simulink model "Tanques_quick_start"  (R2014a)
settings: Solver=ode1  StartTime=0.0  StopTime=200  FixedStep=0.1  RelTol=1e-3
PostLoadFcn:
  | qc_set_target_type(getConfigSet(bdroot, 'QUARC Default Target Configuration'));
values from neighbouring files (symbols this model uses):
  a = sys.a    [Init_SS.m]    (also in test.m)
  b = sys.b    [Init_SS.m]    (also in test.m)
  c = sys.c    [Init_SS.m]    (also in test.m)
  k = [K(2) K(3)]    [Init_SS.m]    (also in test.m = [0.9 0.9])
  ke = K(1)    [Init_SS.m]
  L = acker(a', c', polos_observer)'    [Init_SS.m]    (also in Observer.m = [1.1; 0.2]; test.m = acker(a', c', k)')
undefined symbols (not defined in the file or in its folder): HIL
libraries: quarc_library x3, simulink x1, commrandsrc2 x1
PauseFcn:
  | get_amplitude_and_period(amin, amax, pmin, pmax)
settings Model: SimulationMode=external  ExtModeTrigDuration=30000  Creator=MLevis  LastModifiedBy=Aluno IC
settings SolverCC: PositivePriorityOrder=on
settings DataIOCC: SignalLoggingSaveFormat=ModelDataLogs
settings OptimizationCC: ExpressionDepthLimit=2147483647  InitFltsAndDblsToZero=on
settings DebuggingCC: SaveWithParameterizedLinksMsg=none  UnderspecifiedInitializationDetection=Classic  MultiTaskDSMMsg=warning  MultiTaskCondExecSysMsg=none  FcnCallInpInsideContextMsg=UseLocalSettings  StateNameClashWarn=warning
settings RTWCC: SystemTargetFile=quarc_win64.tlc  TemplateMakefile=quarc_default_tmf  Description=QUARC Win64 Target  ProcessScript=quarc_win64_make_rtw_hook
settings STFCustomTargetCC: CPPClassGenCompliant=on
settings GRTTargetCC: ParMdlRefBuildCompliant=off  CompOptLevelCompliant=off  CombineOutputUpdateFcns=off  MatFileLogging=off  GRTInterface=on  ExtMode=on  ExtModeMexFile=quarc_comm

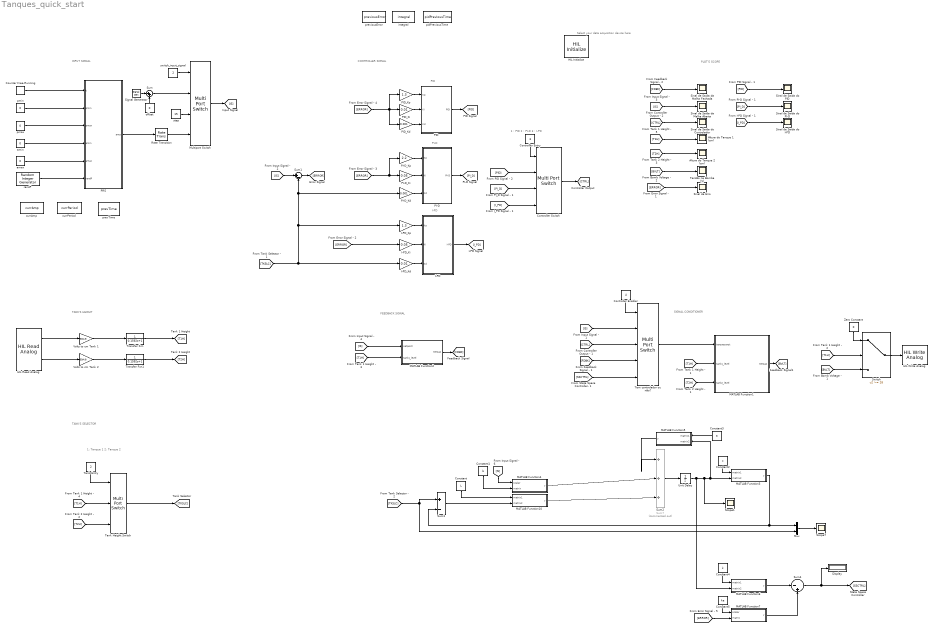
== system Tanques_quick_start ==
  note: INPUT SIGNAL
  note: Select your data acquisition device here
  note: TANK'S HEIGHT
  note: FEEDBACK SIGNAL
  note: CONTROLLER SIGNAL
  note: SIGNAL CONDITIONER
  note: PLOT'S SCOPE
  note: 1 : PID
      | 2 : PI-D
      | 3 : I-PD
  note: I-PD
  note: PI-D
  note: PID
  note: 1: Tanque 1
      | 2: Tanque 2
  note: TANK'S SELECTOR
  Altura do Tanque 1 (cm) : Scope
      settings: TimeRange=200  YMin=-5.5  YMax=30  SaveName=Tank_1_Height_Data
  Altura do Tanque 2 (cm) : Scope
      settings: TimeRange=120  YMin=0  YMax=30  SaveName=Tank_2_Height_Data
  Constant : Constant  Value=L  VectorParams1D=off
  Constant1 : Constant  Value=b  VectorParams1D=off
  Constant2 : Constant  Value=c  VectorParams1D=off
  Constant3 : Constant  Value=a  VectorParams1D=off
  Constant4 : Constant  Value=k  VectorParams1D=off
  Constant5 : Constant  Value=ke  VectorParams1D=off
  "Controller Enabler " : Constant  Value=4
  Controller Entry : Constant  Value=3
  Controller Switch : MultiPortSwitch
  Counter Free-Running : simulink/Sources/Counter Free-Running  NumBits=16  tsamp=1
  Display : Display
  HIL Initialize : quarc_library/Data Acquisition/Generic/Configuration/HIL Initialize  object_name=HIL-1  board_type=q2_usb  board_number=0  board_options=d0=digital;d1=digital;led=auto;update_rate=normal;decimation=1  exclusive=off  active=off  hardware_clocks=[0]  clock_modes=[]  initial_clock_frequencies=[]  set_clock_params_at_start=off  set_clock_params_at_switch_in=off  set_clock_frequencies_at_start=off  set_clock_frequencies_at_switch_in=off  analog_input_channels=[0:1]  analog_input_maximums=10  analog_input_minimums=-10  set_analog_input_params_at_start=on  set_analog_input_params_at_switch_in=off  analog_output_channels=[0:1]  analog_output_maximums=10  analog_output_minimums=-10  initial_analog_outputs=[0]  final_analog_outputs=[0]  watchdog_analog_outputs=0  set_analog_output_params_at_start=on  set_analog_output_params_at_switch_in=off  set_analog_outputs_at_start=on  set_analog_outputs_at_switch_in=off  set_analog_outputs_at_terminate=on  set_analog_outputs_at_switch_out=off  set_analog_outputs_on_watchdog=off  digital_input_channels=[]  digital_output_channels=[]  digital_output_configuration=[]  initial_digital_outputs=[1]  final_digital_outputs=[1]  watchdog_digital_outputs=[1]  set_digital_output_params_at_start=off  set_digital_output_params_at_switch_in=off  set_digital_outputs_at_start=on  set_digital_outputs_at_switch_in=off  set_digital_outputs_at_terminate=on  set_digital_outputs_at_switch_out=off  set_digital_outputs_on_watchdog=off  encoder_channels=[0:1]  quadrature=[4]  encoder_filter_frequency=[]  initial_encoder_counts=[0]  set_encoder_params_at_start=on  set_encoder_params_at_switch_in=off  set_encoder_counts_at_start=on  set_encoder_counts_at_switch_in=off  pwm_channels=[]  pwm_modes=[0]  pwm_frequency=1/0.020  pwm_configuration=[]  pwm_alignment=[]  pwm_polarity=[]  pwm_leading_deadband=[]  pwm_trailing_deadband=[]  initial_pwm_outputs=[0]  final_pwm_outputs=[0]  watchdog_pwm_outputs=[0]  set_pwm_params_at_start=on  set_pwm_params_at_switch_in=off  set_pwm_outputs_at_start=on  set_pwm_outputs_at_switch_in=off  set_pwm_outputs_at_terminate=on  set_pwm_outputs_at_switch_out=off  set_pwm_outputs_on_watchdog=off  other_output_channels=[]  initial_other_outputs=[]  final_other_outputs=[]  watchdog_other_outputs=[]  set_other_outputs_at_start=off  set_other_outputs_at_switch_in=off  set_other_outputs_at_terminate=off  set_other_outputs_at_switch_out=off  set_other_outputs_on_watchdog=off
  HIL Read Analog : quarc_library/Data Acquisition/Generic/Immediate I//O/HIL Read Analog  object_name=HIL-1  channels=[0:1]  sample_time=qc_get_step_size  active=on  vector_output=off
  HIL Write Analog : quarc_library/Data Acquisition/Generic/Immediate I//O/HIL Write Analog  object_name=HIL-1  channels=0  sample_time=-1  active=off  vector_input=off
  I-PD : Subsystem
  I-PD_Kd : Gain  Gain=0.01
  I-PD_Ki : Gain  Gain=0.05
  I-PD_Kp : Gain  Gain=1.3
  MATLAB Function1 : MATLAB Function  TreatAsAtomicUnit=on
  MATLAB Function10 : MATLAB Function  TreatAsAtomicUnit=on
  MATLAB Function2 : MATLAB Function  TreatAsAtomicUnit=on
  MATLAB Function3 : MATLAB Function  TreatAsAtomicUnit=on
  MATLAB Function4 : MATLAB Function  TreatAsAtomicUnit=on
  MATLAB Function5 : MATLAB Function  TreatAsAtomicUnit=on
  MATLAB Function6 : MATLAB Function  TreatAsAtomicUnit=on
  MATLAB Function7 : MATLAB Function  TreatAsAtomicUnit=on
  Multiport Switch : MultiPortSwitch
  Mux : Mux  Inputs=2
  PI-D : Subsystem
  PI-D_Kd : Gain  Gain=0.001
  "PI-D_Ki " : Gain  Gain=0.05
  PI-D_Kp : Gain  Gain=2.2
  PID : Subsystem
  PID_Kd : Gain  Gain=0.001
  PID_Ki : Gain  Gain=0.01
  PID_Kp : Gain  Gain=1.3
  PRS : MATLAB Function  TreatAsAtomicUnit=on
  Rate Transition : RateTransition  OutPortSampleTime=0.1
  Scope1 : Scope
      settings: YMin=0  YMax=50
  Scope7 : Scope
      settings: YMin=0  YMax=50  SaveName=ScopeData6
  Signal Generator : SignalGenerator  Amplitude=15  Frequency=6.2832  Units=rad/sec
  Sinal de Erro : Scope
      settings: TimeRange=200  YMin=-3  YMax=15  SaveName=tensao1
  Sinal de Saída da Malha Aberta : Scope
      settings: TimeRange=200  YMin=9  YMax=15  SaveName=ScopeData3
  Sinal de Saída da Malha Fechada : Scope
      settings: YMin=9.25  YMax=14.75  SaveName=ScopeData7
  Sinal de Saída do Controlador : Scope
      settings: TimeRange=200  YMin=9  YMax=15  SaveName=ScopeData4
  Sinal de Saída do I-PD : Scope
      settings: YMin=-7.5  YMax=32.5  SaveName=I_PD_Data
  Sinal de Saída do PI-D : Scope
      settings: TimeRange=120  YMax=40  SaveName=PI_D_Data
  Sinal de Saída do PID : Scope
      settings: TimeRange=200  YMin=-2.5  YMax=32.5  SaveName=PID_Data
  Sum : Sum  Inputs=|++
  Sum1 : Sum  Inputs=|+-
  Sum2 : Sum  Inputs=|+++
  Sum3 : Sum  Inputs=|+-
  Sum4 : Sum  Inputs=|-+
  Sum7 : Sum  Commented=on  Inputs=|+++
  Switch : Switch  Threshold=28
  Tank Entry : Constant  Value=2
  Tank Height Switch : MultiPortSwitch  Inputs=2
  "Tem controlador ou não? " : MultiPortSwitch  Inputs=4
  Tensão na Bomba (V) : Scope
      settings: TimeRange=30  SaveName=tensao
  Transfer Fcn : TransferFcn  Denominator=[0.1592 1]
  Transfer Fcn1 : TransferFcn  Denominator=[0.1592 1]
  Unit Delay : UnitDelay  SampleTime=-1
  "Volts to cm Tank 1 " : Gain  Gain=30/4.8
  Volts to cm Tank 2 : Gain  Gain=30/4.8
  Zero Constant : Constant  Value=0
  amax : Constant  Value=0  OutDataTypeStr=double
  amin : Constant  Value=0  OutDataTypeStr=double
  currAmp : DataStoreMemory  DataStoreName=currAmp  ReadBeforeWriteMsg=warning  WriteAfterWriteMsg=warning  WriteAfterReadMsg=warning  OutDataTypeStr=double
  currPeriod : DataStoreMemory  DataStoreName=currPeriod  ReadBeforeWriteMsg=warning  WriteAfterWriteMsg=warning  WriteAfterReadMsg=warning  OutDataTypeStr=uint16
  integral : DataStoreMemory  DataStoreName=integral  ReadBeforeWriteMsg=warning  WriteAfterWriteMsg=warning  WriteAfterReadMsg=warning  OutDataTypeStr=double
  offset : Constant  Value=0
  pidPreviousTime : DataStoreMemory  DataStoreName=pidPreviousTime  ReadBeforeWriteMsg=warning  WriteAfterWriteMsg=warning  WriteAfterReadMsg=warning  OutDataTypeStr=double
  pmax : Constant  Value=0  OutDataTypeStr=uint16
  pmin : Constant  Value=0  OutDataTypeStr=uint16
  prevTime : DataStoreMemory  DataStoreName=prevTime  ReadBeforeWriteMsg=warning  WriteAfterWriteMsg=warning  WriteAfterReadMsg=warning  OutDataTypeStr=uint16
  previousError : DataStoreMemory  DataStoreName=previousError  ReadBeforeWriteMsg=warning  WriteAfterWriteMsg=warning  WriteAfterReadMsg=warning  OutDataTypeStr=double
  randP : commrandsrc2/Random Integer Generator  mul=5  seed=37  Ts=1  frameBased=off  sampPerFrame=1  orient=off  outDataType=uint16
  step : Constant  Value=15
  switch_input_signal : Constant  Value=2
  wires:
  HIL Read Analog/1 -> "Volts to cm Tank 1 "/1
  "Volts to cm Tank 1 "/1 -> Transfer Fcn/1
  Transfer Fcn1/1 -> [T2H]
  Volts to cm Tank 2/1 -> Transfer Fcn1/1
  HIL Read Analog/2 -> Volts to cm Tank 2/1
  switch_input_signal/1 -> Multiport Switch/1
  step/1 -> Multiport Switch/3
  Signal Generator/1 -> Sum/1
  offset/1 -> Sum/2
  Sum/1 -> Multiport Switch/2
  Counter Free-Running/1 -> PRS/1(t)
  pmin/1 -> PRS/2(pmin)
  pmax/1 -> PRS/3(pmax)
  amin/1 -> PRS/4(amin)
  amax/1 -> PRS/5(amax)
  randP/1 -> PRS/6(randP)
  PRS/1(amp) -> Rate Transition/1
  Zero Constant/1 -> Switch/1
  Switch/1 -> HIL Write Analog/1
  Rate Transition/1 -> Multiport Switch/4
  Multiport Switch/1 -> [IS]
  Transfer Fcn/1 -> [T1H]
  "Controller Enabler "/1 -> "Tem controlador ou não? "/1
  "Tem controlador ou não? "/1 -> MATLAB Function1/1(tensaoconst)
  [T1H] -> MATLAB Function2/2(tank1_level)
  [T1H] -> MATLAB Function1/2(tank1_level)
  [T1H] -> Switch/2
  [T2H] -> MATLAB Function1/3(tank2_level)
  [IS] -> "Tem controlador ou não? "/2
  [IS] -> Sinal de Saída da Malha Aberta/1
  [IS] -> MATLAB Function2/1(setpoint)
  Controller Switch/1 -> [CTRL]
  [CTRL] -> "Tem controlador ou não? "/3
  MATLAB Function2/1(tensao) -> [FDBK]
  [FDBK] -> "Tem controlador ou não? "/4
  [FDBK] -> Sinal de Saída da Malha Fechada/1
  [T1H] -> Altura do Tanque 1 (cm)/1
  [T2H] -> Altura do Tanque 2 (cm)/1
  MATLAB Function1/1(tensao) -> [BVLT]
  [BVLT] -> Switch/3
  [BVLT] -> Tensão na Bomba (V)/1
  [CTRL] -> Sinal de Saída do Controlador/1
  [ERROR] -> Sinal de Erro/1
  [PID] -> Sinal de Saída do PID/1
  [PI_D] -> Sinal de Saída do PI-D/1
  [I_PD] -> Sinal de Saída do I-PD/1
  PID_Kp/1 -> PID/1(" Kp")
  PID_Kd/1 -> PID/3(Kd)
  PID_Ki/1 -> PID/2(Ki)
  PI-D/1(PI-D) -> [PI_D]
  Sum1/1 -> [ERROR]
  Controller Entry/1 -> Controller Switch/1
  I-PD/1(I-PD) -> [I_PD]
  PID/1(PID) -> [PID]
  [ERROR] -> I-PD_Ki/1
  [ERROR] -> PI-D_Kp/1, "PI-D_Ki "/1
  [ERROR] -> PID_Kd/1, PID_Ki/1, PID_Kp/1
  [PID] -> Controller Switch/2
  [I_PD] -> Controller Switch/4
  [PI_D] -> Controller Switch/3
  PI-D_Kp/1 -> PI-D/1(" Kp")
  PI-D_Kd/1 -> PI-D/3(Kd)
  "PI-D_Ki "/1 -> PI-D/2(" Ki")
  I-PD_Kp/1 -> I-PD/1(" Kp")
  I-PD_Kd/1 -> I-PD/3(Kd)
  I-PD_Ki/1 -> I-PD/2(" Ki")
  [IS] -> Sum1/1
  Constant/1 -> MATLAB Function10/1(matrix1)
  MATLAB Function4/1(y) -> Sum2/2
  [IS] -> MATLAB Function4/1(scalar)
  Constant1/1 -> MATLAB Function4/2(matrix)
  MATLAB Function10/1(y) -> Sum2/3
  MATLAB Function3/1(y) -> Mux/1, Sum3/2
  Constant2/1 -> MATLAB Function3/1(matrix1)
  Constant3/1 -> MATLAB Function5/1(matrix1)
  [TKSLC] -> Mux/2, Sum3/1
  Sum3/1 -> MATLAB Function10/2(matrix2)
  MATLAB Function5/1(y) -> Sum2/1
  Sum2/1 -> Unit Delay/1
  Unit Delay/1 -> MATLAB Function6/2(matrix2), Scope1/1, MATLAB Function3/2(matrix2), MATLAB Function5/2(matrix2)
  Mux/1 -> Scope7/1
  [TKSLC] -> PI-D_Kd/1, Sum1/2, I-PD_Kp/1, I-PD_Kd/1
  Tank Entry/1 -> Tank Height Switch/1
  [T1H] -> Tank Height Switch/2
  [T2H] -> Tank Height Switch/3
  Tank Height Switch/1 -> [TKSLC]
  Constant4/1 -> MATLAB Function6/1(matrix1)
  MATLAB Function6/1(y) -> Sum4/1
  Constant5/1 -> MATLAB Function7/1(scalar)
  MATLAB Function7/1(y) -> Sum4/2
  [ERROR] -> MATLAB Function7/2(matrix)
  Sum4/1 -> Display/1, [SSCTRL]
  [SSCTRL] -> "Tem controlador ou não? "/5

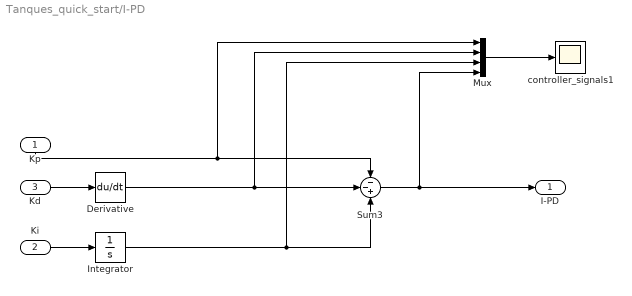
== system Tanques_quick_start/I-PD ==
  " Kp" : Inport
  " Ki" : Inport  Port=2
  Kd : Inport  Port=3
  Derivative : Derivative
  Integrator : Integrator  LimitOutput=on  UpperSaturationLimit=35  LowerSaturationLimit=-1
  Mux : Mux
  Sum3 : Sum  Inputs=--+
  controller_signals1 : Scope
      settings: ShowLegends=on  TimeRange=200  YMin=-10  YMax=150
  I-PD : Outport
  wires:
  Derivative/1 -> Mux/2, Sum3/2
  " Kp"/1 -> Mux/1, Sum3/1
  Sum3/1 -> Mux/4, I-PD/1
  Integrator/1 -> Mux/3, Sum3/3
  Kd/1 -> Derivative/1
  " Ki"/1 -> Integrator/1
  Mux/1 -> controller_signals1/1

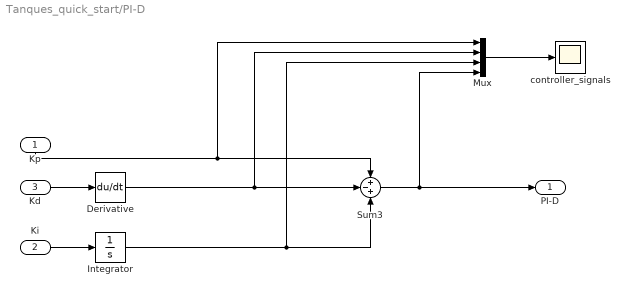
== system Tanques_quick_start/PI-D ==
  " Kp" : Inport
  " Ki" : Inport  Port=2
  Kd : Inport  Port=3
  Derivative : Derivative
  Integrator : Integrator
  Mux : Mux
  Sum3 : Sum  Inputs=+-+
  controller_signals : Scope
      settings: ShowLegends=on  TimeRange=150  YMin=-15  YMax=50
  PI-D : Outport
  wires:
  Derivative/1 -> Mux/2, Sum3/2
  " Kp"/1 -> Mux/1, Sum3/1
  Sum3/1 -> Mux/4, PI-D/1
  Integrator/1 -> Mux/3, Sum3/3
  Kd/1 -> Derivative/1
  " Ki"/1 -> Integrator/1
  Mux/1 -> controller_signals/1

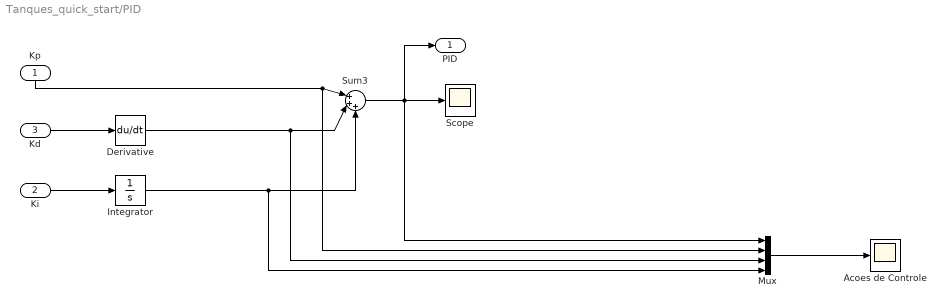
== system Tanques_quick_start/PID ==
  " Kp" : Inport
  Ki : Inport  Port=2
  Kd : Inport  Port=3
  Acoes de Controle : Scope
      settings: ShowLegends=on  TimeRange=200  YMin=-2.5  YMax=32.5  SaveName=ScopeData5
  Derivative : Derivative
  Integrator : Integrator  LimitOutput=on
  Mux : Mux
  Scope : Scope
      settings: ShowLegends=on  TimeRange=90  YMin=10  YMax=47.5  SaveName=ScopeData2
  Sum3 : Sum  Inputs=|+++
  PID : Outport
  wires:
  Derivative/1 -> Mux/3, Sum3/2
  Integrator/1 -> Mux/4, Sum3/3
  " Kp"/1 -> Mux/2, Sum3/1
  Ki/1 -> Integrator/1
  Kd/1 -> Derivative/1
  Sum3/1 -> Mux/1, PID/1, Scope/1
  Mux/1 -> Acoes de Controle/1

== matlab function Tanques_quick_start/MATLAB Function1 ==
  data: tensaoconst input; tensao output; tank1_level input; tank2_level input
function tensao  = trava(tensaoconst, tank1_level, tank2_level)
%#codegen
%Trava para a tensão

if(tensaoconst > 4)
   tensaoconst = 4;
elseif(tensaoconst < -4)
    tensaoconst = -4;
end

%%Trava pro tanque
hmax = 30;

if(tank1_level < 2 && tensaoconst < 0)
    tensaoconst=0;
elseif(-tank1_level+hmax > 5 && -tank1_level+hmax < 6)
    tensaoconst=tensaoconst;
elseif(-tank1_level+hmax > 4 && -tank1_level+hmax < 5)
    tensaoconst=tensaoconst*0.9;
elseif(-tank1_level+hmax > 3 && -tank1_level+hmax < 4)
    tensaoconst=tensaoconst*0.8;
elseif(-tank1_level+hmax > 2 && -tank1_level+hmax< 3)
    tensaoconst=tensaoconst*0.79;
elseif(-tank1_level+hmax > 1 && -tank1_level+hmax < 1.5)
    tensaoconst=tensaoconst*0.70;
elseif(-tank1_level+hmax > 0.5 && -tank1_level+hmax < 0.8)
    tensaoconst=tensaoconst*0.55;
end

tensao = tensaoconst;

== matlab function Tanques_quick_start/PRS ==
  data: t input; pmin input; pmax input; amp output; amin input; amax input; randP input; currAmp data_store_memory; currPeriod data_store_memory; prevTime data_store_memory
function amp = fcn(t, pmin, pmax, amin, amax, randP)
    global currPeriod;
    global currAmp;
    global prevTime;    
    if(t - prevTime >= currPeriod)        
        if(randP + pmin < pmax)
            currPeriod = pmin + randP;
        else
            currPeriod = randP;
        end
        [currAmp, x] = get_amplitude_and_period(amin, amax, 1, 3);
        prevTime = t;
    end
    amp = currAmp;    
end

== matlab function Tanques_quick_start/MATLAB Function2 ==
  data: setpoint input; tensao output; tank1_level input
function tensao  = fcn(setpoint, tank1_level)
%#codegen
if(setpoint > 30)
    setpoint = 30;
elseif(setpoint < 0)
    setpoint = 0;
end
tensao = setpoint - tank1_level;
end

== matlab function Tanques_quick_start/MATLAB Function10 ==
  data: matrix1 input; y output; matrix2 input
function y = M_x_M(matrix1, matrix2)
y = matrix_x_matrix(matrix1, matrix2);

== matlab function Tanques_quick_start/MATLAB Function3 ==
  data: matrix1 input; y output; matrix2 input
function y = M_x_M(matrix1, matrix2)
y = matrix_x_matrix(matrix1, matrix2);

== matlab function Tanques_quick_start/MATLAB Function4 ==
  data: scalar input; y output; matrix input
function y = S_x_M(scalar, matrix)
y = scalar_x_matrix(scalar, matrix);

== matlab function Tanques_quick_start/MATLAB Function5 ==
  data: matrix1 input; y output; matrix2 input
function y = M_x_M(matrix1, matrix2)
y = matrix_x_matrix(matrix1, matrix2);

== matlab function Tanques_quick_start/MATLAB Function6 ==
  data: matrix1 input; y output; matrix2 input
function y = M_x_M(matrix1, matrix2)
y = matrix_x_matrix(matrix1, matrix2);

== matlab function Tanques_quick_start/MATLAB Function7 ==
  data: scalar input; y output; matrix input
function y = S_x_M(scalar, matrix)
y = scalar_x_matrix(scalar, matrix);
